simulink model "A1"  (R2023b)
settings: Solver=FixedStepAuto  StartTime=0.0  StopTime=10.0  FixedStep=1e-3  RelTol=1e-3  EnableMultiTasking=on
settings Model: ExtModeTrigDuration=5  Creator=Bernic  LastModifiedBy=Bernic
settings OptimizationCC: EnhancedBackFolding=on  PassReuseOutputArgsAs=Individual arguments  ZeroExternalMemoryAtStartup=off  ZeroInternalMemoryAtStartup=off  MaxStackSize=64  OptimizeBlockOrder=speed  DifferentSizesBufferReuse=on  OptimizationCustomize=off  EfficientTunableParamExpr=on
settings DebuggingCC: ParameterTunabilityLossMsg=error
settings HardwareCC: ProdBitPerPointer=32  ProdBitPerSizeT=32  ProdBitPerPtrDiffT=32  ProdLargestAtomicInteger=Long  ProdLargestAtomicFloat=Double  ProdWordSize=32  ProdHWDeviceType=ARM Compatible->ARM Cortex
settings SFSimCC: MATLABDynamicMemAlloc=off
settings RTWCC: Description=Embedded Coder  SystemTargetFile=ert.tlc  HardwareBoard=NXP FRDM-K64F  TLCOptions="-aInlineSetEventsForThisBaseRateFcn=TLC_FALSE -aSuppressMultiTaskScheduler=TLC_FALSE  -aRateBasedStepFcn=0"  TemplateMakefile=ert_default_tmf  Toolchain=GNU Tools for ARM Embedded Processors
settings CodeAppCC: ForceParamTrailComments=on  IgnoreCustomStorageClasses=off  OperatorAnnotations=on  SimulinkDataObjDesc=on  SFDataObjDesc=on  InsertBlockDesc=on
settings ERTTargetCC: ExtModeTransport=4  ExtModeMexFile=sendToCommService

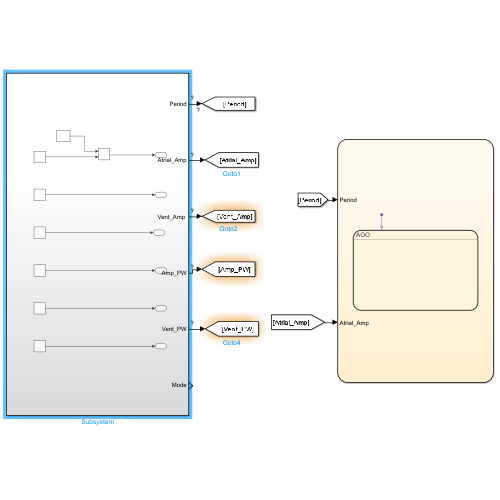
[thumbnail: Simulink's stored preview of the top-level diagram]
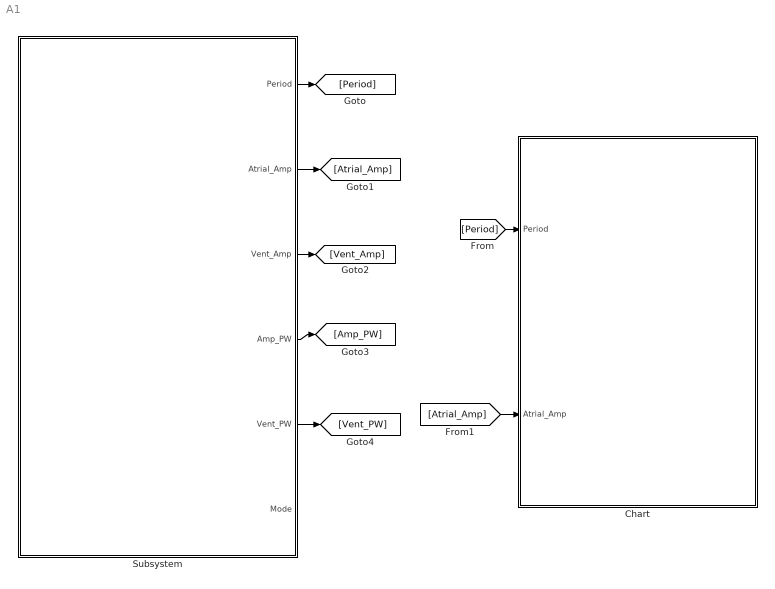
== system A1 ==
  Chart : Stateflow chart  TreatAsAtomicUnit=on
  Subsystem : Subsystem
  wires:
  Subsystem/1(Period) -> [Period]
  [Period] -> Chart/1(Period)
  Subsystem/2(Atrial_Amp) -> [Atrial_Amp]
  [Atrial_Amp] -> Chart/2(Atrial_Amp)
  Subsystem/3("Vent_Amp ") -> [Vent_Amp]
  Subsystem/4(Amp_PW) -> [Amp_PW]
  Subsystem/5(Vent_PW) -> [Vent_PW]

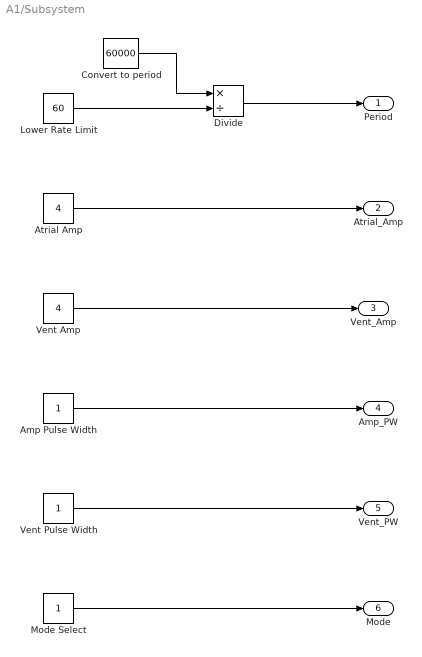
== system A1/Subsystem ==
  Amp Pulse Width : Constant
  Atrial Amp : Constant  Value=4
  Convert to period : Constant  Value=60000  VectorParams1D=off
  Divide : Product  Inputs=*/
  Lower Rate Limit : Constant  Value=60  VectorParams1D=off
  Mode Select : Constant  VectorParams1D=off
  Vent Amp : Constant  Value=4
  Vent Pulse Width : Constant  VectorParams1D=off
  Period : Outport
  Atrial_Amp : Outport  Port=2
  "Vent_Amp " : Outport  Port=3
  Amp_PW : Outport  Port=4
  Vent_PW : Outport  Port=5
  Mode : Outport  Port=6
  wires:
  Lower Rate Limit/1 -> Divide/2
  Atrial Amp/1 -> Atrial_Amp/1
  Vent Amp/1 -> "Vent_Amp "/1
  Amp Pulse Width/1 -> Amp_PW/1
  Vent Pulse Width/1 -> Vent_PW/1
  Divide/1 -> Period/1
  Convert to period/1 -> Divide/1
  Mode Select/1 -> Mode/1

== stateflow chart A1/Chart ==
  state AOO
    state Charging
      entry:
      % Charging C22
      ATR_PACE_CTRL = 0
      VENT_PACE_CTRL = 0
      PACING_REF_PWM = Atrial_Amp
      PACE_CHARGE_CTRL = 1
      %  Discharge C21 while
      PACE_GND_CTRL = 1
      ATR_PACE_CTRL = 0
      Z_ATR_CTRL = 0
      Z_VENT_CTRL = 0
      ATR_GND_CTRL = 0
      VENT_GND_CTRL = 0
      VENT_PACE_CTRL = 0
    state Pacing
      entry:
      % Discharging C22 to C21
      PACE_CHARGE_CTRL = 0
      PACE_GND_CTRL = 1
      VENT_PACE_CTRL = 0
      Z_ATR_CTRL = 0
      Z_VENT_CTRL = 0
      ATR_PACE_CTRL = 0
      ATR_GND_CTRL = 1
      VENT_GND_CTRL = 0
    (default) -> Charging
    Pacing -> Charging : [after(period - atr_pw, msec)]
    Charging -> Pacing : [after(atr_pw, msec)]
  (default) -> AOO
  data: Period input; Atrial_Amp input
